simulink model "PID_ciagly"  (R2021a)
settings: Solver=VariableStepAuto  StartTime=0.0  StopTime=100.0  RelTol=1e-3
values from neighbouring files (symbols this model uses):
  Kp = 0.222    [PID_ciagly_params.m]
  Td = 2.4144    [PID_ciagly_params.m]    (also in PID_dysrk.m; Zadanie2.m = 0; Zadanie6_PID.m)
  Ti = 10.06    [PID_ciagly_params.m]    (also in PID_dysrk.m; Zadanie2.m = 0; Zadanie6_PID.m)
settings Model: Creator=ADMIN  LastModifiedBy=ADMIN

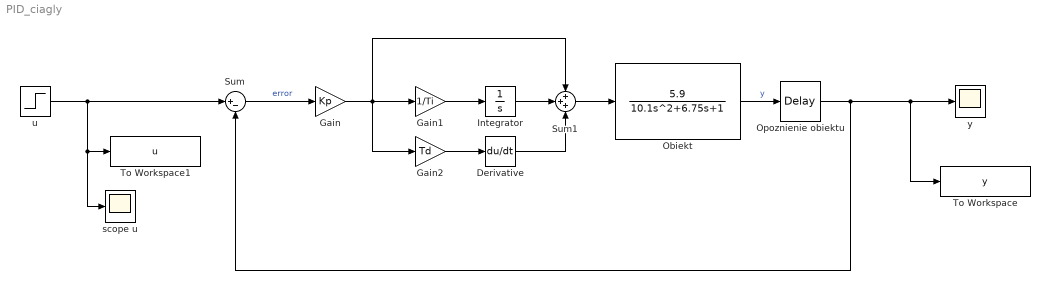
== system PID_ciagly ==
  " Opoznienie obiektu" : TransportDelay  DelayTime=5
  " Obiekt" : TransferFcn  Numerator=[5.9]  Denominator=[10.1 6.75 1]
  Derivative : Derivative
  Gain : Gain  Gain=Kp
  Gain1 : Gain  Gain=1/Ti
  Gain2 : Gain  Gain=Td
  Integrator : Integrator
  Sum : Sum  Inputs=|+-
  Sum1 : Sum  Inputs=+++
  To Workspace : ToWorkspace  VariableName=y  SaveFormat=Structure With Time  SampleTime=-1
  To Workspace1 : ToWorkspace  VariableName=u  SaveFormat=Structure With Time  SampleTime=-1
  scope u : Scope
  u : Step  SampleTime=0
  y : Scope
  wires:
  u/1 -> scope u/1, To Workspace1/1, Sum/1
  Sum/1 -> Gain/1  "error"
  Gain2/1 -> Derivative/1
  Gain1/1 -> Integrator/1
  Gain/1 -> Gain1/1, Sum1/1, Gain2/1
  Integrator/1 -> Sum1/2
  Derivative/1 -> Sum1/3
  Sum1/1 -> " Obiekt"/1
  " Obiekt"/1 -> " Opoznienie obiektu"/1  "y"
  " Opoznienie obiektu"/1 -> Sum/2, To Workspace/1, y/1
